simulink model "extractLocal_ros"  (R2024a)
settings: Solver=FixedStepAuto  StartTime=0.0  StopTime=10.0  RelTol=1e-3
InitFcn:
  | % Make sure server is running
  | svrMdlName = 'localMapServer';
  | load_system(svrMdlName);
  | set_param(svrMdlName,'SimulationCommand','Start');
  | pause(1);
StopFcn:
  | % Make sure server is running
  | svrMdlName = 'localMapServer';
  | load_system(svrMdlName);
  | set_param(svrMdlName,'SimulationCommand','Stop');
model workspace (MAT data in the model file):
  SL_ROS_VariableLengthArrays_MaxSizes.CommonInfo.ArrayTruncateAction = 'EmitWarning'
  SL_ROS_VariableLengthArrays_MaxSizes.MsgTypeMap = containers.Map
  SL_ROS_VariableLengthArrays_MaxSizes.MsgTypeMap.serialization.keys = {'std_msgs/Int8MultiArray'}
  SL_ROS_VariableLengthArrays_MaxSizes.MsgTypeMap.serialization.values{1}.PropertyName = 'data'
  SL_ROS_VariableLengthArrays_MaxSizes.MsgTypeMap.serialization.values{1}.DataType = 'int8'
  SL_ROS_VariableLengthArrays_MaxSizes.MsgTypeMap.serialization.values{1}.MaxLength = 1500000
  SL_ROS_VariableLengthArrays_MaxSizes.MsgTypeMap.serialization.uniformity = 0
  SL_ROS_VariableLengthArrays_MaxSizes.MsgTypeMap.serialization.keyType = 'char'
  SL_ROS_VariableLengthArrays_MaxSizes.MsgTypeMap.serialization.valueType = 'any'
undefined symbols (not defined in the file): curpose, lookaheadtime, maxvelocity, tuneableTEBParams, worldgridloc, worldGridLoc, worldmat, worldMat, worldRes, worldresolution
libraries: roshelperlib x3, ros2lib x2
settings Model: Creator=cstabile  LastModifiedBy=cstabile
settings OptimizationCC: EnhancedBackFolding=on  PassReuseOutputArgsAs=Individual arguments  ZeroExternalMemoryAtStartup=off  ZeroInternalMemoryAtStartup=off  MaxStackSize=64  OptimizeBlockOrder=speed  DifferentSizesBufferReuse=on  OptimizationCustomize=off  EfficientTunableParamExpr=on
settings DebuggingCC: ParameterTunabilityLossMsg=error
settings SFSimCC: MATLABDynamicMemAlloc=off
settings RTWCC: Description=Embedded Coder  SystemTargetFile=ert.tlc  HardwareBoard=Robot Operating System 2 (ROS 2)  TLCOptions="-aInlineSetEventsForThisBaseRateFcn=TLC_FALSE -aSuppressMultiTaskScheduler=TLC_FALSE  -aRateBasedStepFcn=0"  TemplateMakefile=ert_default_tmf  Toolchain=Colcon Tools  TargetLang=C++
settings CodeAppCC: ForceParamTrailComments=on  IgnoreCustomStorageClasses=off  OperatorAnnotations=on  SimulinkDataObjDesc=on  SFDataObjDesc=on  InsertBlockDesc=on
settings ERTTargetCC: CodeInterfacePackaging=C++ class  RootIOFormat=Structure reference

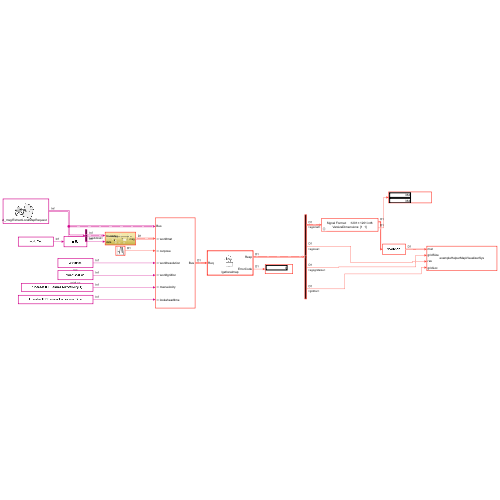
[thumbnail: Simulink's stored preview of the top-level diagram]
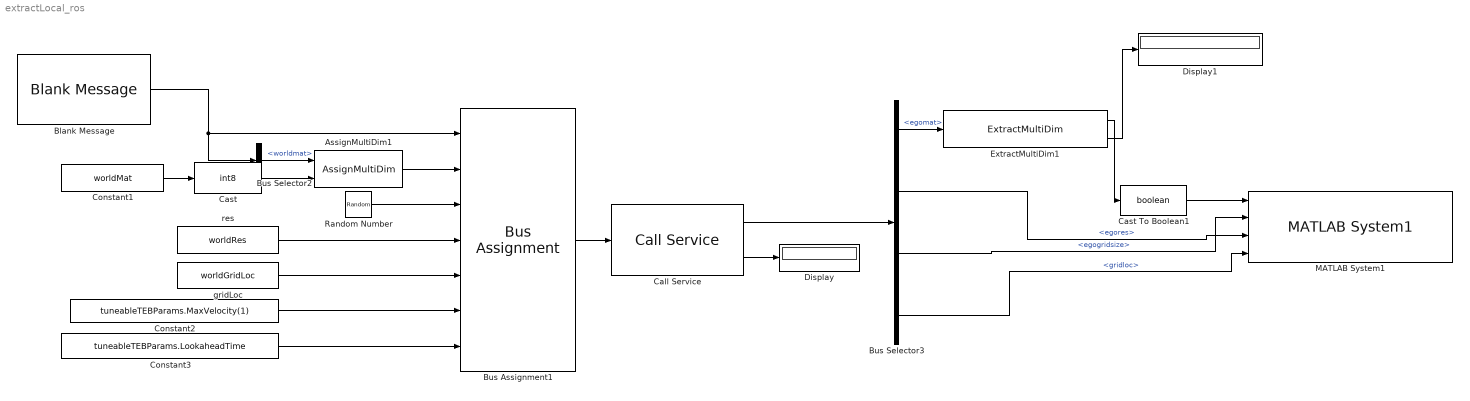
== system extractLocal_ros ==
  AssignMultiDim1 : roshelperlib/AssignMultiDim  SystemSampleTime=-1  VariantActivationTime=update diagram  AllowFlexibleInterface=on  Latency=0  AutoFrameSizeCalculation=off
  Blank Message : ros2lib/Blank Message  messageClass=Service Request  entityType=offroad_msg/ExtractLocalMap  messageType=offroad_msg/ExtractLocalMapRequest  SampleTime=inf
  Bus Assignment1 : BusAssignment  AssignedSignals=worldmat,curpose,worldresolution,worldgridloc,maxvelocity,lookaheadtime
  Bus Selector2 : BusSelector  OutputSignals=worldmat
  Bus Selector3 : BusSelector  OutputSignals=egomat,egores,egogridsize,gridloc
  Call Service : ros2lib/Call Service  topicSource=Specify your own  service=/getlocalmap  serviceType=offroad_msg/ExtractLocalMap  connectionTimeout=.2  ShowErrorCodeOutput=on  legacyBusStruct=off  QOSHistory=Keep last  QOSDepth=1  QOSReliability=Reliable  QOSDurability=Volatile  QOSDeadline=Inf  QOSLifespan=Inf  QOSLiveliness=Automatic  QOSLeaseDuration=Inf  QOSAvoidROSNamespaceConventions=off
  Cast : DataTypeConversion  OutDataTypeStr=int8  SaturateOnIntegerOverflow=off  RndMeth=Floor
  Cast To Boolean1 : DataTypeConversion  OutDataTypeStr=boolean  SaturateOnIntegerOverflow=off  RndMeth=Floor
  Constant1 : Constant  Value=worldMat
  Constant2 : Constant  Value=tuneableTEBParams.MaxVelocity(1)
  Constant3 : Constant  Value=tuneableTEBParams.LookaheadTime
  Display : Display
  Display1 : Display
  ExtractMultiDim1 : roshelperlib/ExtractMultiDim  userDataType=int8  dims=[1201 1201]  isVarsize=on  varsizeDims=[1 1]  returnFixedTF=off
  MATLAB System1 : roshelperlib/MATLAB System1  MapType=SDF  DisplayVisual=on  SimulateUsing=Interpreted execution
  Random Number : RandomNumber  Mean=[500 500 0]  Variance=[100 100 0]  SampleTime=.2
  gridLoc : Constant  Value=worldGridLoc  VectorParams1D=off
  res : Constant  Value=worldRes
  wires:
  Blank Message/1 -> Bus Selector2/1, Bus Assignment1/1
  Constant1/1 -> Cast/1
  Bus Selector2/1 -> AssignMultiDim1/1  "<worldmat>"
  Bus Assignment1/1 -> Call Service/1
  Call Service/1 -> Bus Selector3/1
  Call Service/2 -> Display/1
  Bus Selector3/1 -> ExtractMultiDim1/1  "<egomat>"
  ExtractMultiDim1/1 -> Cast To Boolean1/1
  ExtractMultiDim1/2 -> Display1/1
  Cast To Boolean1/1 -> MATLAB System1/1
  Cast/1 -> AssignMultiDim1/2
  Bus Selector3/4 -> MATLAB System1/4  "<gridloc>"
  Random Number/1 -> Bus Assignment1/3
  AssignMultiDim1/1 -> Bus Assignment1/2
  res/1 -> Bus Assignment1/4
  gridLoc/1 -> Bus Assignment1/5
  Constant2/1 -> Bus Assignment1/6
  Constant3/1 -> Bus Assignment1/7
  Bus Selector3/3 -> MATLAB System1/2  "<egogridsize>"
  Bus Selector3/2 -> MATLAB System1/3  "<egores>"
